simulink model "mod_firmware_NVH_v6"  (R2022a)
settings: Solver=FixedStepDiscrete  StartTime=0.0  StopTime=Inf  RelTol=1e-3  EnableMultiTasking=on
InitFcn:
  | params_NVH;
undefined symbols (not defined in the file): denz, DiscIntNeverNeededParam, Down, GPTRIP1SEL, GPTRIP2SEL, KiTs, Kp, numz, POS, rate_lim, target, Tper, Tref, Ts, TZ1, TZ2, Up
libraries: simulink x10, hdlsllib x7, mcbcontrolslib x5, c2802xlib x4, c2837xDlib x4, c280xlib x2, c2000lib x1, slpidlib x1
(part 1 of 2)
settings Model: ExtModeTrigDuration=8  Creator=Renato  LastModifiedBy=Renato
settings SolverCC: AlgebraicLoopSolver=TrustRegion  AutoInsertRateTranBlk=on
settings OptimizationCC: DefaultUnderspecifiedDataType=single  EnhancedBackFolding=on  PassReuseOutputArgsAs=Individual arguments  MaxStackSize=1024  OptimizeBlockOrder=speed  DifferentSizesBufferReuse=on  OptimizationCustomize=off  DenormalBehavior=FlushToZero  EfficientTunableParamExpr=on
settings DebuggingCC: MultiTaskDSMMsg=none  ParameterPrecisionLossMsg=none  ParameterTunabilityLossMsg=error  UnconnectedInputMsg=warning  UnconnectedOutputMsg=warning  UnconnectedLineMsg=warning  SFMachineParentedDataDiag=warning
settings HardwareCC: ProdBitPerChar=16  ProdBitPerInt=16  ProdBitPerPointer=32  ProdBitPerSizeT=32  ProdBitPerPtrDiffT=32  ProdLargestAtomicInteger=Integer  ProdLargestAtomicFloat=None  ProdWordSize=16  ProdLongLongMode=on  ProdHWDeviceType=Texas Instruments->C2000
settings SFSimCC: MATLABDynamicMemAlloc=off
settings RTWCC: SystemTargetFile=ert.tlc  HardwareBoard=TI Delfino F28379D LaunchPad  TemplateMakefile=ert_default_tmf  Toolchain=Texas Instruments Code Composer Studio (C2000)  DLArmComputeVersion=19.05
settings CodeAppCC: ForceParamTrailComments=on  IgnoreCustomStorageClasses=off  OperatorAnnotations=on  SimulinkDataObjDesc=on  SFDataObjDesc=on  InsertBlockDesc=on
settings ERTTargetCC: CodeReplacementLibrary=TI C28x  ExtModeStaticAllocSize=10000

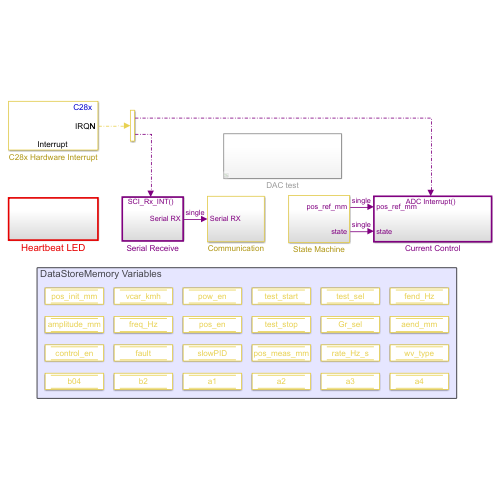
[thumbnail: Simulink's stored preview of the top-level diagram]
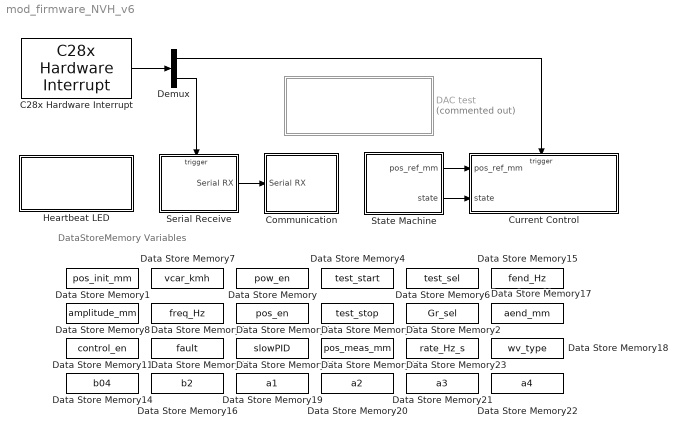
== system mod_firmware_NVH_v6 ==
  note: DataStoreMemory Variables
  C28x Hardware Interrupt : c2000lib/Scheduling/C28x Hardware Interrupt  irqnumbers=[1 9]  pienumbers=[2 1]  irqpriorities=[30 50]  irqpreempts=[1 0]  showinput=off  dspchiptype=C280X
      settings: SourceProductBaseCode=TIC2000
  Communication : Subsystem
  Current Control : Subsystem
  DAC test : Subsystem  Commented=on
  Data Store Memory : DataStoreMemory  DataStoreName=pow_en  ReadBeforeWriteMsg=warning  WriteAfterWriteMsg=warning  WriteAfterReadMsg=warning  ShowAdditionalParam=off
  Data Store Memory1 : DataStoreMemory  DataStoreName=pos_init_mm  ReadBeforeWriteMsg=warning  WriteAfterWriteMsg=warning  WriteAfterReadMsg=warning  ShowAdditionalParam=off
  Data Store Memory10 : DataStoreMemory  DataStoreName=fault  ReadBeforeWriteMsg=warning  WriteAfterWriteMsg=warning  WriteAfterReadMsg=warning  ShowAdditionalParam=off
  Data Store Memory11 : DataStoreMemory  DataStoreName=control_en  ReadBeforeWriteMsg=warning  WriteAfterWriteMsg=warning  WriteAfterReadMsg=warning  ShowAdditionalParam=off
  Data Store Memory12 : DataStoreMemory  DataStoreName=slowPID  ReadBeforeWriteMsg=warning  WriteAfterWriteMsg=warning  WriteAfterReadMsg=warning  ShowAdditionalParam=off
  Data Store Memory13 : DataStoreMemory  DataStoreName=pos_meas_mm  ReadBeforeWriteMsg=warning  WriteAfterWriteMsg=warning  WriteAfterReadMsg=warning  ShowAdditionalParam=off
  Data Store Memory14 : DataStoreMemory  DataStoreName=b04  ReadBeforeWriteMsg=warning  WriteAfterWriteMsg=warning  WriteAfterReadMsg=warning  ShowAdditionalParam=off
  Data Store Memory15 : DataStoreMemory  DataStoreName=fend_Hz  ReadBeforeWriteMsg=warning  WriteAfterWriteMsg=warning  WriteAfterReadMsg=warning  ShowAdditionalParam=off
  Data Store Memory16 : DataStoreMemory  DataStoreName=b2  ReadBeforeWriteMsg=warning  WriteAfterWriteMsg=warning  WriteAfterReadMsg=warning  ShowAdditionalParam=off
  Data Store Memory17 : DataStoreMemory  DataStoreName=aend_mm  ReadBeforeWriteMsg=warning  WriteAfterWriteMsg=warning  WriteAfterReadMsg=warning  ShowAdditionalParam=off
  Data Store Memory18 : DataStoreMemory  DataStoreName=wv_type  ReadBeforeWriteMsg=warning  WriteAfterWriteMsg=warning  WriteAfterReadMsg=warning  ShowAdditionalParam=off
  Data Store Memory19 : DataStoreMemory  DataStoreName=a1  ReadBeforeWriteMsg=warning  WriteAfterWriteMsg=warning  WriteAfterReadMsg=warning  ShowAdditionalParam=off
  Data Store Memory2 : DataStoreMemory  DataStoreName=Gr_sel  ReadBeforeWriteMsg=warning  WriteAfterWriteMsg=warning  WriteAfterReadMsg=warning  ShowAdditionalParam=off
  Data Store Memory20 : DataStoreMemory  DataStoreName=a2  ReadBeforeWriteMsg=warning  WriteAfterWriteMsg=warning  WriteAfterReadMsg=warning  ShowAdditionalParam=off
  Data Store Memory21 : DataStoreMemory  DataStoreName=a3  ReadBeforeWriteMsg=warning  WriteAfterWriteMsg=warning  WriteAfterReadMsg=warning  ShowAdditionalParam=off
  Data Store Memory22 : DataStoreMemory  DataStoreName=a4  ReadBeforeWriteMsg=warning  WriteAfterWriteMsg=warning  WriteAfterReadMsg=warning  ShowAdditionalParam=off
  Data Store Memory23 : DataStoreMemory  DataStoreName=rate_Hz_s  ReadBeforeWriteMsg=warning  WriteAfterWriteMsg=warning  WriteAfterReadMsg=warning  ShowAdditionalParam=off
  Data Store Memory3 : DataStoreMemory  DataStoreName=pos_en  ReadBeforeWriteMsg=warning  WriteAfterWriteMsg=warning  WriteAfterReadMsg=warning  ShowAdditionalParam=off
  Data Store Memory4 : DataStoreMemory  DataStoreName=test_start  ReadBeforeWriteMsg=warning  WriteAfterWriteMsg=warning  WriteAfterReadMsg=warning  ShowAdditionalParam=off
  Data Store Memory5 : DataStoreMemory  DataStoreName=test_stop  ReadBeforeWriteMsg=warning  WriteAfterWriteMsg=warning  WriteAfterReadMsg=warning  ShowAdditionalParam=off
  Data Store Memory6 : DataStoreMemory  DataStoreName=test_sel  ReadBeforeWriteMsg=warning  WriteAfterWriteMsg=warning  WriteAfterReadMsg=warning  ShowAdditionalParam=off
  Data Store Memory7 : DataStoreMemory  DataStoreName=vcar_kmh  ReadBeforeWriteMsg=warning  WriteAfterWriteMsg=warning  WriteAfterReadMsg=warning  ShowAdditionalParam=off
  Data Store Memory8 : DataStoreMemory  DataStoreName=amplitude_mm  ReadBeforeWriteMsg=warning  WriteAfterWriteMsg=warning  WriteAfterReadMsg=warning  ShowAdditionalParam=off
  Data Store Memory9 : DataStoreMemory  DataStoreName=freq_Hz  ReadBeforeWriteMsg=warning  WriteAfterWriteMsg=warning  WriteAfterReadMsg=warning  ShowAdditionalParam=off
  Demux : Demux  Outputs=2
  Heartbeat LED : Subsystem  TreatAsAtomicUnit=on
  Serial Receive : Subsystem  SystemSampleTime=1e-3
  State Machine : Subsystem
  wires:
  C28x Hardware Interrupt/1 -> Demux/1
  Demux/2 -> Serial Receive/Trigger
  Demux/1 -> Current Control/Trigger
  Serial Receive/1(Serial RX) -> Communication/1(Serial RX)
  State Machine/1(pos_ref_mm) -> Current Control/1(pos_ref_mm)
  State Machine/2(state) -> Current Control/2(state)

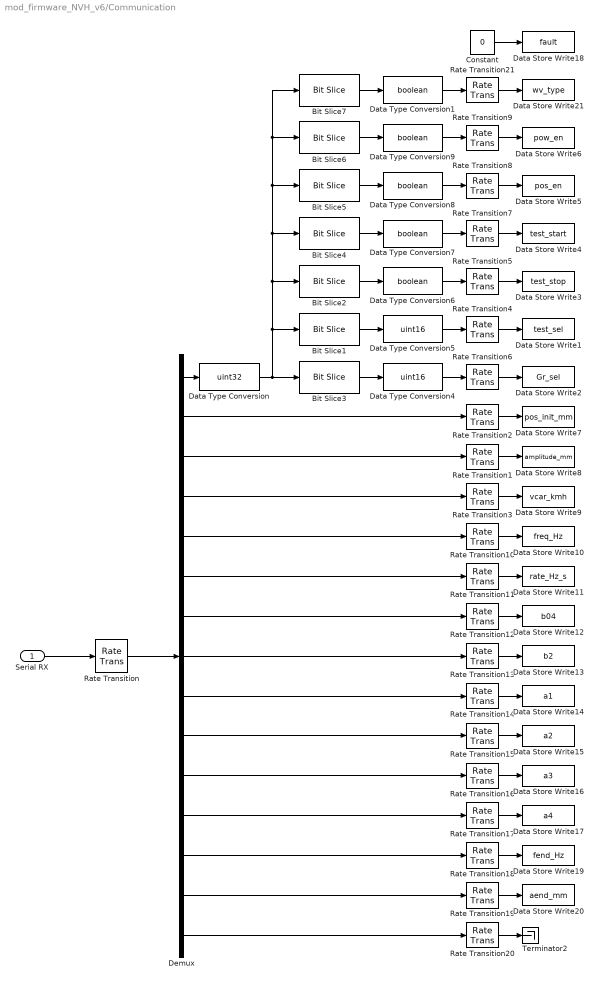
== system mod_firmware_NVH_v6/Communication ==
  Serial RX : Inport
  Bit Slice1 : hdlsllib/Logic and Bit Operations/Bit Slice  lidx=3  ridx=2
      settings: SourceProductBaseCode=SL
  Bit Slice2 : hdlsllib/Logic and Bit Operations/Bit Slice  lidx=4  ridx=4
      settings: SourceProductBaseCode=SL
  Bit Slice3 : hdlsllib/Logic and Bit Operations/Bit Slice  lidx=1  ridx=0
      settings: SourceProductBaseCode=SL
  Bit Slice4 : hdlsllib/Logic and Bit Operations/Bit Slice  lidx=5  ridx=5
      settings: SourceProductBaseCode=SL
  Bit Slice5 : hdlsllib/Logic and Bit Operations/Bit Slice  lidx=6  ridx=6
      settings: SourceProductBaseCode=SL
  Bit Slice6 : hdlsllib/Logic and Bit Operations/Bit Slice  lidx=7  ridx=7
      settings: SourceProductBaseCode=SL
  Bit Slice7 : hdlsllib/Logic and Bit Operations/Bit Slice  lidx=8  ridx=8
      settings: SourceProductBaseCode=SL
  Constant : Constant  Value=0  OutDataTypeStr=boolean  SampleTime=Ts
  Data Store Write1 : DataStoreWrite  DataStoreName=test_sel  IndexOptions=Index vector (dialog)  Indices=1  OutputSizes=1
  Data Store Write10 : DataStoreWrite  DataStoreName=freq_Hz  IndexOptions=Index vector (dialog)  Indices=1  OutputSizes=1
  Data Store Write11 : DataStoreWrite  DataStoreName=rate_Hz_s  IndexOptions=Index vector (dialog)  Indices=1  OutputSizes=1
  Data Store Write12 : DataStoreWrite  DataStoreName=b04  IndexOptions=Index vector (dialog)  Indices=1  OutputSizes=1
  Data Store Write13 : DataStoreWrite  DataStoreName=b2  IndexOptions=Index vector (dialog)  Indices=1  OutputSizes=1
  Data Store Write14 : DataStoreWrite  DataStoreName=a1  IndexOptions=Index vector (dialog)  Indices=1  OutputSizes=1
  Data Store Write15 : DataStoreWrite  DataStoreName=a2  IndexOptions=Index vector (dialog)  Indices=1  OutputSizes=1
  Data Store Write16 : DataStoreWrite  DataStoreName=a3  IndexOptions=Index vector (dialog)  Indices=1  OutputSizes=1
  Data Store Write17 : DataStoreWrite  DataStoreName=a4  IndexOptions=Index vector (dialog)  Indices=1  OutputSizes=1
  Data Store Write18 : DataStoreWrite  DataStoreName=fault  IndexOptions=Index vector (dialog)  Indices=1  OutputSizes=1
  Data Store Write19 : DataStoreWrite  DataStoreName=fend_Hz  IndexOptions=Index vector (dialog)  Indices=1  OutputSizes=1
  Data Store Write2 : DataStoreWrite  DataStoreName=Gr_sel  IndexOptions=Index vector (dialog)  Indices=1  OutputSizes=1
  Data Store Write20 : DataStoreWrite  DataStoreName=aend_mm  IndexOptions=Index vector (dialog)  Indices=1  OutputSizes=1
  Data Store Write21 : DataStoreWrite  DataStoreName=wv_type  IndexOptions=Index vector (dialog)  Indices=1  OutputSizes=1
  Data Store Write3 : DataStoreWrite  DataStoreName=test_stop  IndexOptions=Index vector (dialog)  Indices=1  OutputSizes=1
  Data Store Write4 : DataStoreWrite  DataStoreName=test_start  IndexOptions=Index vector (dialog)  Indices=1  OutputSizes=1
  Data Store Write5 : DataStoreWrite  DataStoreName=pos_en  IndexOptions=Index vector (dialog)  Indices=1  OutputSizes=1
  Data Store Write6 : DataStoreWrite  DataStoreName=pow_en  IndexOptions=Index vector (dialog)  Indices=1  OutputSizes=1
  Data Store Write7 : DataStoreWrite  DataStoreName=pos_init_mm  IndexOptions=Index vector (dialog)  Indices=1  OutputSizes=1
  Data Store Write8 : DataStoreWrite  DataStoreName=amplitude_mm  IndexOptions=Index vector (dialog)  Indices=1  OutputSizes=1
  Data Store Write9 : DataStoreWrite  DataStoreName=vcar_kmh  IndexOptions=Index vector (dialog)  Indices=1  OutputSizes=1
  Data Type Conversion : DataTypeConversion  OutDataTypeStr=uint32  ConvertRealWorld=Stored Integer (SI)  SaturateOnIntegerOverflow=off  RndMeth=Floor
  Data Type Conversion{1,6..9} (5 alike) : DataTypeConversion  OutDataTypeStr=boolean  RndMeth=Simplest  SaturateOnIntegerOverflow=off
  Data Type Conversion4 : DataTypeConversion  OutDataTypeStr=uint16  RndMeth=Simplest  SaturateOnIntegerOverflow=off
  Data Type Conversion5 : DataTypeConversion  OutDataTypeStr=uint16  RndMeth=Simplest  SaturateOnIntegerOverflow=off
  Demux : Demux  Outputs=15
  Rate Transition : RateTransition  Deterministic=off  InitialCondition=zeros(15,1)  OutPortSampleTime=Ts
  Rate Transition{1..21} (21 alike) : RateTransition  Deterministic=off
  Terminator2 : Terminator
  wires:
  Rate Transition/1 -> Demux/1
  Serial RX/1 -> Rate Transition/1
  Demux/1 -> Data Type Conversion/1
  Bit Slice3/1 -> Data Type Conversion4/1
  Data Type Conversion4/1 -> Rate Transition6/1
  Bit Slice1/1 -> Data Type Conversion5/1
  Data Type Conversion5/1 -> Rate Transition4/1
  Data Type Conversion6/1 -> Rate Transition5/1
  Bit Slice2/1 -> Data Type Conversion6/1
  Data Type Conversion7/1 -> Rate Transition7/1
  Bit Slice4/1 -> Data Type Conversion7/1
  Data Type Conversion8/1 -> Rate Transition8/1
  Bit Slice5/1 -> Data Type Conversion8/1
  Data Type Conversion9/1 -> Rate Transition9/1
  Bit Slice6/1 -> Data Type Conversion9/1
  Rate Transition6/1 -> Data Store Write2/1
  Rate Transition4/1 -> Data Store Write1/1
  Rate Transition5/1 -> Data Store Write3/1
  Rate Transition7/1 -> Data Store Write4/1
  Rate Transition8/1 -> Data Store Write5/1
  Rate Transition9/1 -> Data Store Write6/1
  Demux/2 -> Rate Transition2/1
  Rate Transition2/1 -> Data Store Write7/1
  Rate Transition1/1 -> Data Store Write8/1
  Demux/3 -> Rate Transition1/1
  Rate Transition3/1 -> Data Store Write9/1
  Demux/4 -> Rate Transition3/1
  Demux/5 -> Rate Transition10/1
  Rate Transition10/1 -> Data Store Write10/1
  Constant/1 -> Data Store Write18/1
  Rate Transition20/1 -> Terminator2/1
  Rate Transition19/1 -> Data Store Write20/1
  Rate Transition18/1 -> Data Store Write19/1
  Rate Transition17/1 -> Data Store Write17/1
  Demux/6 -> Rate Transition11/1
  Rate Transition11/1 -> Data Store Write11/1
  Rate Transition13/1 -> Data Store Write13/1
  Rate Transition15/1 -> Data Store Write15/1
  Rate Transition12/1 -> Data Store Write12/1
  Rate Transition14/1 -> Data Store Write14/1
  Rate Transition16/1 -> Data Store Write16/1
  Demux/7 -> Rate Transition12/1
  Demux/8 -> Rate Transition13/1
  Demux/9 -> Rate Transition14/1
  Demux/10 -> Rate Transition15/1
  Demux/11 -> Rate Transition16/1
  Demux/14 -> Rate Transition19/1
  Demux/12 -> Rate Transition17/1
  Demux/15 -> Rate Transition20/1
  Demux/13 -> Rate Transition18/1
  Data Type Conversion/1 -> Bit Slice5/1, Bit Slice7/1, Bit Slice6/1, Bit Slice4/1, Bit Slice2/1, Bit Slice1/1, Bit Slice3/1
  Rate Transition21/1 -> Data Store Write21/1
  Data Type Conversion1/1 -> Rate Transition21/1
  Bit Slice7/1 -> Data Type Conversion1/1

== system mod_firmware_NVH_v6/Current Control ==
  pos_ref_mm : Inport
  state : Inport  Port=2
  ADC Interrupt : TriggerPort  TriggerType=function-call  VariantControl=Variant
  ADC sampling : Subsystem
      settings: PortSchema="{\"entries\":[{\"content\":{\"sides\":[{\"content\":{\"connectorIds\":[]},\"type\":\"ConnectorPlacement.EquallySpacedRectSide\",\"uuid\":\"7a2cf5f2-16d9-4c06-9e50-766569fc1ffb\"},{\"content\":{\"connectorIds\":[],\"side\":\"RIGHT\"},\"type\":\"ConnectorPlacement.EquallySpacedRectSide\",\"uuid\":\"bcd2dcb7-1f81-4f8a-ab4d-3b7c4b9f9b31\"},{\"content\":{\"connectorIds\":[\"Out1\",\"In1\"],\"side\":\"TOP\"},\"type\":\"ConnectorPlacement.EquallySpacedRectSide\",\"uuid\":\"ccc507c4-0562-40ca-8656-7bb2ecd7cc5f\"}]},\"type\":\"ConnectorPlacement.EquallySpacedConnector\",\"uuid\":\"1a99524b-495c-42f0-b183-14d68da7a393\"}],\"packageUris\":[\"http://schema.mathworks.com/mf0/Connector/R2020b\"],\"version\":\"1.0\"}"
  Data Serial Output : Subsystem
  Duty conditioning : Subsystem
      settings: PortSchema="{\"entries\":[{\"content\":{\"sides\":[{\"content\":{\"connectorIds\":[\"In1\"]},\"type\":\"ConnectorPlacement.EquallySpacedRectSide\",\"uuid\":\"a0799500-10a4-4433-8e57-709958199fd5\"},{\"content\":{\"connectorIds\":[\"Out1\",\"In2\"],\"side\":\"RIGHT\"},\"type\":\"ConnectorPlacement.EquallySpacedRectSide\",\"uuid\":\"3bf72f91-b298-49c1-8116-d920c6c6ec77\"},{\"content\":{\"connectorIds\":[],\"side\":\"TOP\"},\"type\":\"ConnectorPlacement.EquallySpacedRectSide\",\"uuid\":\"802670f8-b9dd-4762-928c-43325713460b\"}]},\"type\":\"ConnectorPlacement.EquallySpacedConnector\",\"uuid\":\"a1eb57ea-35c4-47bc-baa8-d00685cc87f7\"}],\"packageUris\":[\"http://schema.mathworks.com/mf0/Connector/R2020b\"],\"version\":\"1.0\"}"
  Hardware Initialization : Subsystem
  Mux : Mux  Inputs=3
  PWM : Subsystem
  wires:
  Duty conditioning/1(dutyA) -> PWM/1(dutyA), ADC sampling/1(dutyA)
  Mux/1 -> Data Serial Output/1(send_vec)
  state/1 -> Mux/3
  pos_ref_mm/1 -> Mux/1, Duty conditioning/1(pos_ref_mm)
  ADC sampling/1(pos_meas) -> Duty conditioning/2(pos_meas), Mux/2

== system mod_firmware_NVH_v6/DAC test ==
  DAC : c2837xDlib/DAC  channel=B  saturate=on
      settings: SourceProductBaseCode=TIC2000
  Data Type Conversion : DataTypeConversion  OutDataTypeStr=uint16  SaturateOnIntegerOverflow=off  RndMeth=Floor
  Sine Wave : Sin  Amplitude=2048-100  Bias=2048  Frequency=2*pi  SampleTime=Ts
  Sine Wave1 : Sin  Amplitude=100  Frequency=2*pi*2000  SampleTime=Ts
  Sum : Sum  Inputs=|++
  wires:
  Data Type Conversion/1 -> DAC/1
  Sum/1 -> Data Type Conversion/1
  Sine Wave/1 -> Sum/1
  Sine Wave1/1 -> Sum/2

== system mod_firmware_NVH_v6/Heartbeat LED ==
  Data Store Read1 : DataStoreRead  DataStoreName=pos_en  IndexOptions=Index vector (dialog)  Indices=1  OutputSizes=1
  Digital Output : c2837xDlib/Digital Output  GPIO_Number=GPIO32~GPIO39  GPIO_Bit0=off  GPIO_BIT0_Toggle=on  GPIO_Bit1=off  GPIO_BIT1_Toggle=off  GPIO_Bit2=on  GPIO_BIT2_Toggle=off  GPIO_Bit3=off  GPIO_BIT3_Toggle=off  GPIO_Bit4=off  GPIO_BIT4_Toggle=off  GPIO_Bit5=off  GPIO_BIT5_Toggle=off  GPIO_Bit6=off  GPIO_BIT6_Toggle=off  GPIO_Bit7=off  GPIO_BIT7_Toggle=off
      settings: SourceProductBaseCode=TIC2000
  wires:
  Data Store Read1/1 -> Digital Output/1

== system mod_firmware_NVH_v6/Serial Receive ==
  SCI_Rx_INT : TriggerPort  TriggerType=function-call  VariantControl=Variant
  SCI Receive : c280xlib/SCI Receive  sciModule=A  dataHead=''  headerCheckMaxCount=16  dataTail=''  dataType=single  dataLenOptions=Length via dialog  dataDim=15  maxDataLength=1  initValue=0  errOption=Output the last received value  errValue=0  sampleTime=-1  blockingMode=on  timeOut=0.00875  outputStatus=off
      settings: SourceProductBaseCode=TIC2000
  Serial RX : Outport  VectorParamsAs1DForOutWhenUnconnected=off
  wires:
  SCI Receive/1 -> Serial RX/1

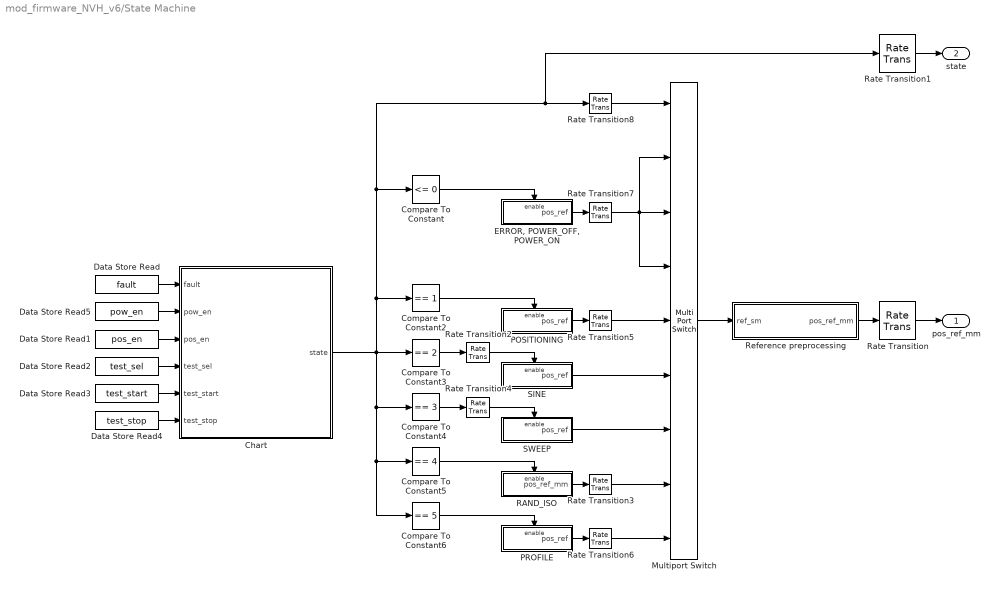
== system mod_firmware_NVH_v6/State Machine ==
  Chart : Stateflow chart  TreatAsAtomicUnit=on
  Compare To Constant : simulink/Logic and Bit Operations/Compare To Constant  relop=<=  const=0  OutDataTypeStr=boolean
  Compare To Constant2 : simulink/Logic and Bit Operations/Compare To Constant  relop===  const=1  OutDataTypeStr=boolean
  Compare To Constant3 : simulink/Logic and Bit Operations/Compare To Constant  relop===  const=2  OutDataTypeStr=boolean
  Compare To Constant4 : simulink/Logic and Bit Operations/Compare To Constant  relop===  const=3  OutDataTypeStr=boolean
  Compare To Constant5 : simulink/Logic and Bit Operations/Compare To Constant  relop===  const=4  OutDataTypeStr=boolean
  Compare To Constant6 : simulink/Logic and Bit Operations/Compare To Constant  relop===  const=5  OutDataTypeStr=boolean
  Data Store Read : DataStoreRead  DataStoreName=fault  SampleTime=Tref  IndexOptions=Index vector (dialog)  Indices=1  OutputSizes=1
  Data Store Read1 : DataStoreRead  DataStoreName=pos_en  SampleTime=Tref  IndexOptions=Index vector (dialog)  Indices=1  OutputSizes=1
  Data Store Read2 : DataStoreRead  DataStoreName=test_sel  SampleTime=Tref  IndexOptions=Index vector (dialog)  Indices=1  OutputSizes=1
  Data Store Read3 : DataStoreRead  DataStoreName=test_start  SampleTime=Tref  IndexOptions=Index vector (dialog)  Indices=1  OutputSizes=1
  Data Store Read4 : DataStoreRead  DataStoreName=test_stop  SampleTime=Tref  IndexOptions=Index vector (dialog)  Indices=1  OutputSizes=1
  Data Store Read5 : DataStoreRead  DataStoreName=pow_en  SampleTime=Tref  IndexOptions=Index vector (dialog)  Indices=1  OutputSizes=1
  "ERROR, POWER_OFF, POWER_ON" : Subsystem  TreatAsAtomicUnit=on
  Multiport Switch : MultiPortSwitch  DataPortOrder=Specify indices  Inputs=7  DataPortIndices={-2,-1,0,1,2,3,4,5}  SaturateOnIntegerOverflow=off  InputSameDT=off
  POSITIONING : Subsystem  TreatAsAtomicUnit=on
  PROFILE : Subsystem  TreatAsAtomicUnit=on
  RAND_ISO : Subsystem  TreatAsAtomicUnit=on
  Rate Transition : RateTransition  Deterministic=off
  Rate Transition1 : RateTransition  Deterministic=off
  Rate Transition{2..8} (7 alike) : RateTransition  Deterministic=off  OutPortSampleTime=Tper
  Reference preprocessing : Subsystem
  SINE : Subsystem  TreatAsAtomicUnit=on
  SWEEP : Subsystem  TreatAsAtomicUnit=on
  pos_ref_mm : Outport
  state : Outport  Port=2
  wires:
  Data Store Read3/1 -> Chart/5(test_start)
  Data Store Read2/1 -> Chart/4(test_sel)
  Data Store Read/1 -> Chart/1(fault)
  Data Store Read1/1 -> Chart/3(pos_en)
  Data Store Read4/1 -> Chart/6(test_stop)
  Compare To Constant/1 -> "ERROR, POWER_OFF, POWER_ON"/Enable
  "ERROR, POWER_OFF, POWER_ON"/1(pos_ref) -> Rate Transition7/1
  Compare To Constant2/1 -> POSITIONING/Enable
  Compare To Constant6/1 -> PROFILE/Enable
  Compare To Constant5/1 -> RAND_ISO/Enable
  Compare To Constant4/1 -> Rate Transition4/1
  Compare To Constant3/1 -> Rate Transition2/1
  Rate Transition1/1 -> state/1
  Rate Transition/1 -> pos_ref_mm/1
  Chart/1(state) -> Rate Transition1/1, Rate Transition8/1, Compare To Constant/1, Compare To Constant2/1, Compare To Constant4/1, Compare To Constant6/1, Compare To Constant5/1, Compare To Constant3/1
  Data Store Read5/1 -> Chart/2(pow_en)
  POSITIONING/1(pos_ref) -> Rate Transition5/1
  RAND_ISO/1(pos_ref_mm) -> Rate Transition3/1
  PROFILE/1(pos_ref) -> Rate Transition6/1
  Multiport Switch/1 -> Reference preprocessing/1(ref_sm)
  Reference preprocessing/1(pos_ref_mm) -> Rate Transition/1
  Rate Transition2/1 -> SINE/Enable
  SINE/1(pos_ref) -> Multiport Switch/6
  Rate Transition4/1 -> SWEEP/Enable
  SWEEP/1(pos_ref) -> Multiport Switch/7
  Rate Transition6/1 -> Multiport Switch/9
  Rate Transition3/1 -> Multiport Switch/8
  Rate Transition5/1 -> Multiport Switch/5
  Rate Transition7/1 -> Multiport Switch/4, Multiport Switch/2, Multiport Switch/3
  Rate Transition8/1 -> Multiport Switch/1

== system mod_firmware_NVH_v6/Current Control/ADC sampling ==
  dutyA : Inport
  Convert : Subsystem
  H1-J7 64 : c2802xlib/ADC  blkParamProc=C2000_Type4  ADCModule=C  samplingMode=Single sample mode  ADCResolution=12-bit (Single-ended input)  useSOC1=SOC1  useSOC2=SOC0_SOC1  SOCAcquisitionWindow=300  SOCTriggerSource=ePWM1_ADCSOCA  SOCInterruptTrigger=No ADCINT  Ts=-1  dType=uint16  postInterrupt=off  interruptSel=ADCINT1  ADCINTContinuous=on  endma=off  chdma=1  conv1=ADCINA0  conv2=ADCINA0 and ADCINB0  conv1_Type4=ADCIN5  conv2_Type4=ADCIN0 and ADCIN1
  IIR Filter : mcbcontrolslib/IIR Filter  VariantControl=Low Pass Filter  VariantSelect=Low-pass  Filter_constant=0.12  advancedSettings=on  Ts=Ts  cutOff_freq=434.0589
      settings: SourceProductBaseCode=MT
  ISENA : c2802xlib/ADC  blkParamProc=C2000_Type4  ADCModule=B  samplingMode=Single sample mode  ADCResolution=12-bit (Single-ended input)  useSOC1=SOC0  useSOC2=SOC0_SOC1  SOCAcquisitionWindow=300  SOCTriggerSource=ePWM1_ADCSOCA  SOCInterruptTrigger=No ADCINT  Ts=-1  dType=uint16  postInterrupt=on  interruptSel=ADCINT1  ADCINTContinuous=on  endma=off  chdma=1  conv1=ADCINA0  conv2=ADCINA0 and ADCINB0  conv1_Type4=ADCIN2  conv2_Type4=ADCIN0 and ADCIN1
  Terminator : Terminator
  Terminator1 : Terminator
  pos_meas : Outport  InitialOutput=0  VectorParamsAs1DForOutWhenUnconnected=off
  wires:
  H1-J7 64/1 -> Convert/1(ADC)
  dutyA/1 -> Terminator/1
  ISENA/1 -> Terminator1/1
  Convert/1(mm) -> IIR Filter/1
  IIR Filter/1 -> pos_meas/1

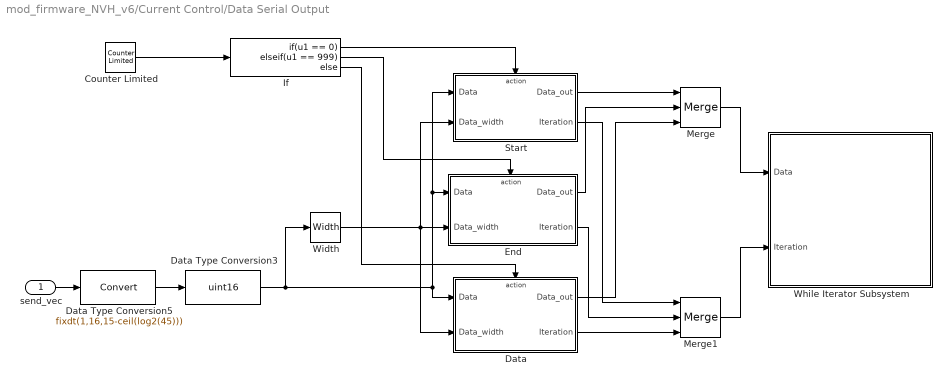
== system mod_firmware_NVH_v6/Current Control/Data Serial Output ==
  send_vec : Inport
  Counter Limited : simulink/Sources/Counter Limited  uplimit=999  tsamp=-1
  Data : Subsystem  TreatAsAtomicUnit=on
  Data Type Conversion3 : DataTypeConversion  OutDataTypeStr=uint16  ConvertRealWorld=Stored Integer (SI)  SaturateOnIntegerOverflow=off  RndMeth=Floor
  Data Type Conversion5 : DataTypeConversion  OutDataTypeStr=fixdt(1,16,15-ceil(log2(45)))  RndMeth=Simplest  SaturateOnIntegerOverflow=off
  End : Subsystem  TreatAsAtomicUnit=on
  If : If  IfExpression=u1 == 0  ElseIfExpressions=u1 == 999
  Merge : Merge  Inputs=3
  Merge1 : Merge  Inputs=3
  Start : Subsystem  TreatAsAtomicUnit=on
  While Iterator Subsystem : Subsystem  TreatAsAtomicUnit=on
  Width : Width  OutDataTypeMode=All ports same datatype  DataType=uint16
  wires:
  Merge/1 -> While Iterator Subsystem/1(Data)
  If/2 -> End/Action
  If/3 -> Data/Action
  Counter Limited/1 -> If/1
  End/1(Data_out) -> Merge/2
  Width/1 -> Start/2(Data_width), Data/2(Data_width), End/2(Data_width)
  Start/1(Data_out) -> Merge/1
  Start/2(Iteration) -> Merge1/1
  Merge1/1 -> While Iterator Subsystem/2(Iteration)
  Data/1(Data_out) -> Merge/3
  If/1 -> Start/Action
  End/2(Iteration) -> Merge1/2
  Data/2(Iteration) -> Merge1/3
  Data Type Conversion3/1 -> Width/1, Start/1(Data), End/1(Data), Data/1(Data)
  send_vec/1 -> Data Type Conversion5/1
  Data Type Conversion5/1 -> Data Type Conversion3/1

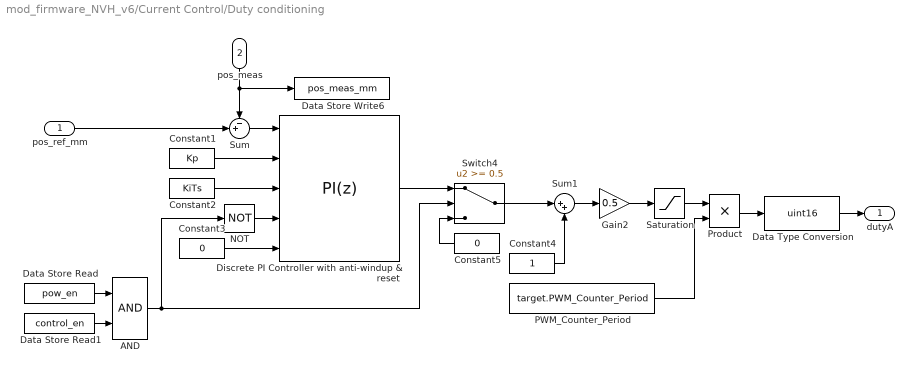
== system mod_firmware_NVH_v6/Current Control/Duty conditioning ==
  pos_ref_mm : Inport
  pos_meas : Inport  Port=2
  AND : Logic  IconShape=distinctive  AllPortsSameDT=off  OutDataTypeStr=boolean
  Constant1 : Constant  Value=Kp  OutDataTypeStr=dataType  SampleTime=-1
  Constant2 : Constant  Value=KiTs  OutDataTypeStr=dataType  SampleTime=-1
  Constant3 : Constant  Value=0  OutDataTypeStr=dataType  SampleTime=-1
  Constant4 : Constant  OutDataTypeStr=dataType  SampleTime=-1
  Constant5 : Constant  Value=0  OutDataTypeStr=dataType  SampleTime=-1
  Data Store Read : DataStoreRead  DataStoreName=pow_en  IndexOptions=Index vector (dialog)  Indices=1  OutputSizes=1
  Data Store Read1 : DataStoreRead  DataStoreName=control_en  IndexOptions=Index vector (dialog)  Indices=1  OutputSizes=1
  Data Store Write6 : DataStoreWrite  DataStoreName=pos_meas_mm  IndexOptions=Index vector (dialog)  Indices=1  OutputSizes=1
  Data Type Conversion : DataTypeConversion  OutDataTypeStr=uint16  RndMeth=Simplest
  Discrete PI Controller with anti-windup & reset : slpidlib/PID Controller  Controller=PI  Form=Parallel  TimeDomain=Discrete-time  UseExternalTs=off  SampleTime=-1  IntegratorMethod=Forward Euler  FilterMethod=Forward Euler  ControllerParametersSource=external  P=1  I=1  UseKiTs=on  D=0  N=100  UseFilter=on  TunerSelectOption=Transfer Function Based (PID Tuner App)  InitialConditionSource=external  InitialConditionForIntegrator=0  InitialConditionForFilter=0  DifferentiatorICPrevScaledInput=0  ExternalReset=level  TrackingMode=off  Kt=1  LimitOutput=on  SatLimitsSource=internal  UpperSaturationLimit=1  LowerSaturationLimit=-1  LinearizeAsGain=on  AntiWindupMode=clamping  Kb=1  RndMeth=Simplest  POutMin=[]  POutMax=[]  IOutMin=[]  IOutMax=[]  DOutMin=[]  DOutMax=[]  NOutMin=[]  NOutMax=[]  SumOutMin=[]  SumOutMax=[]  SaturationOutDataTypeStr=Inherit: Inherit via back propagation  SaturationOutMin=[]  SaturationOutMax=[]  PParamMin=[]  PParamMax=[]  IParamMin=[]  IParamMax=[]  DParamMin=[]  DParamMax=[]  NParamMin=[]  NParamMax=[]  KbParamMin=[]  KbParamMax=[]  KtParamMin=[]  KtParamMax=[]  KbOutMin=[]  KbOutMax=[]  KtOutMin=[]  KtOutMax=[]  IntegratorOutMin=[]  IntegratorOutMax=[]  FilterOutMin=[]  FilterOutMax=[]  SumI1OutMin=[]  SumI1OutMax=[]  SumI2OutMin=[]  SumI2OutMax=[]  SumI3OutMin=[]  SumI3OutMax=[]  SumI4OutMin=[]  SumI4OutMax=[]  SumDOutMin=[]  SumDOutMax=[]  DifferentiatorOutMin=[]  DifferentiatorOutMax=[]  FilterDiffOutCoefMin=[]  FilterDiffOutCoefMax=[]  ReciprocalOutMin=[]  ReciprocalOutMax=[]  SumDenOutMin=[]  SumDenOutMax=[]  SumNumOutMin=[]  SumNumOutMax=[]  DivideOutMin=[]  DivideOutMax=[]  UdiffTsProdOutMin=[]  UdiffTsProdOutMax=[]  NTsProdOutMin=[]  NTsProdOutMax=[]  UintegralTsProdOutMin=[]  UintegralTsProdOutMax=[]  UngainTsProdOutMin=[]  UngainTsProdOutMax=[]  ClampingZeroOutDataTypeStr=Inherit: Inherit via back propagation  ClampingZeroOutMin=[]  ClampingZeroOutMax=[]  FilterDenConstantOutDataTypeStr=Inherit: Inherit via back propagation  FilterDenConstantOutMin=[]  FilterDenConstantOutMax=[]  PCopyOutDataTypeStr=Inherit: Inherit via back propagation  PCopyOutMin=[]  PCopyOutMax=[]  NCopyOutDataTypeStr=Inherit: Inherit via back propagation  NCopyOutMin=[]  NCopyOutMax=[]  IntegratorContinuousStateAttributes=''  IntegratorStateMustResolveToSignalObject=off  IntegratorRTWStateStorageClass=Auto  FilterContinuousStateAttributes=''  FilterStateMustResolveToSignalObject=off  FilterRTWStateStorageClass=Auto  ParallelPVariant=ExternalParameters  IdealPVariant=Disabled  IVariant=ExternalParameters  DVariant=Disabled  IntegratorVariant=Discrete  SatVariant=Enabled  AWVariant=DiscClampingParallel  PCopyVariant=Disabled  TRVariant=Disabled  FdbkBlocksVariant=Forward  IdealPFdbkVariant=Disabled  SatFdbkVariant=Disabled  DerivativeFilterVariant=Disabled  NVariant=Disabled  NCopyVariant=Disabled_SignalSpec  FilterICVariant=Disabled  IntegratorICVariant=ExternalICs  ExternalResetVariant=ExternalReset  TRSumVariant=Passthrough  SumFdbkVariant=Disabled  SumVariant=Sum_PI  TsampFilterVariant=InternalTs  TsampNgainVariant=Passthrough  TsampIntegralVariant=Passthrough  ExternalSaturationOutDataTypeStr=Inherit: Same as second input  aMode=5
  Gain2 : Gain  Gain=0.5  OutDataTypeStr=dataType  RndMeth=Simplest
  NOT : Logic  Operator=NOT  IconShape=distinctive  AllPortsSameDT=off  OutDataTypeStr=boolean
  PWM_Counter_Period : Constant  Value=target.PWM_Counter_Period  OutDataTypeStr=dataType  SampleTime=-1
  Product : Product  RndMeth=Simplest  OutDataTypeStr=Inherit: Same as first input
  Saturation : Saturate  UpperLimit=0.71  LowerLimit=0.29  RndMeth=Simplest
  Sum : Sum  Inputs=-+|
  Sum1 : Sum  Inputs=|++
  Switch4 : Switch  Threshold=0.5  RndMeth=Simplest  SaturateOnIntegerOverflow=off  InputSameDT=off
  dutyA : Outport
  wires:
  Product/1 -> Data Type Conversion/1
  PWM_Counter_Period/1 -> Product/2
  Data Type Conversion/1 -> dutyA/1
  pos_ref_mm/1 -> Sum/2
  pos_meas/1 -> Data Store Write6/1, Sum/1
  Sum/1 -> Discrete PI Controller with anti-windup & reset/1
  Constant4/1 -> Sum1/2
  Sum1/1 -> Gain2/1
  Gain2/1 -> Saturation/1
  Saturation/1 -> Product/1
  AND/1 -> NOT/1, Switch4/2
  NOT/1 -> Discrete PI Controller with anti-windup & reset/4
  Constant3/1 -> Discrete PI Controller with anti-windup & reset/5
  Discrete PI Controller with anti-windup & reset/1 -> Switch4/1
  Switch4/1 -> Sum1/1
  Constant5/1 -> Switch4/3
  Data Store Read/1 -> AND/1
  Data Store Read1/1 -> AND/2
  Constant1/1 -> Discrete PI Controller with anti-windup & reset/2
  Constant2/1 -> Discrete PI Controller with anti-windup & reset/3

== system mod_firmware_NVH_v6/Current Control/Hardware Initialization ==
  " Grounding the SPI clock for the DRV8323" : c2837xDlib/Digital Output  GPIO_Number=GPIO56~GPIO63  GPIO_Bit0=off  GPIO_BIT0_Toggle=off  GPIO_Bit1=off  GPIO_BIT1_Toggle=off  GPIO_Bit2=off  GPIO_BIT2_Toggle=off  GPIO_Bit3=off  GPIO_BIT3_Toggle=off  GPIO_Bit4=on  GPIO_BIT4_Toggle=off  GPIO_Bit5=off  GPIO_BIT5_Toggle=off  GPIO_Bit6=off  GPIO_BIT6_Toggle=off  GPIO_Bit7=off  GPIO_BIT7_Toggle=off
      settings: SourceProductBaseCode=TIC2000
  Constant : Constant  Value=0  OutDataTypeStr=uint16  SampleTime=-1
  DRV8323 Enable : c2837xDlib/Digital Output  GPIO_Number=GPIO64~GPIO71  GPIO_Bit0=off  GPIO_BIT0_Toggle=off  GPIO_Bit1=off  GPIO_BIT1_Toggle=off  GPIO_Bit2=off  GPIO_BIT2_Toggle=off  GPIO_Bit3=on  GPIO_BIT3_Toggle=off  GPIO_Bit4=off  GPIO_BIT4_Toggle=off  GPIO_Bit5=off  GPIO_BIT5_Toggle=off  GPIO_Bit6=off  GPIO_BIT6_Toggle=off  GPIO_Bit7=off  GPIO_BIT7_Toggle=off
      settings: SourceProductBaseCode=TIC2000
  Data Store Read : DataStoreRead  DataStoreName=pow_en  IndexOptions=Index vector (dialog)  Indices=1  OutputSizes=1
  wires:
  Constant/1 -> " Grounding the SPI clock for the DRV8323"/1
  Data Store Read/1 -> DRV8323 Enable/1

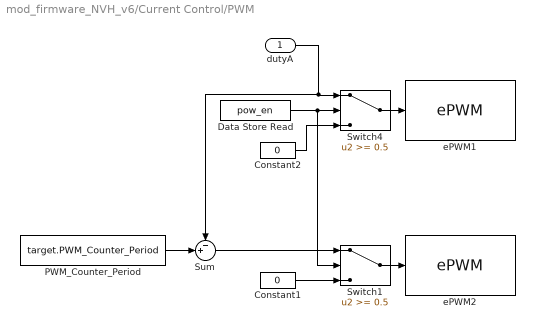
== system mod_firmware_NVH_v6/Current Control/PWM ==
  dutyA : Inport
  Constant1 : Constant  Value=0  OutDataTypeStr=uint16
  Constant2 : Constant  Value=0  OutDataTypeStr=uint16
  Data Store Read : DataStoreRead  DataStoreName=pow_en  IndexOptions=Index vector (dialog)  Indices=1  OutputSizes=1
  PWM_Counter_Period : Constant  Value=target.PWM_Counter_Period  OutDataTypeStr=uint16  SampleTime=-1
  Sum : Sum  Inputs=-+|
  Switch1 : Switch  Threshold=0.5  RndMeth=Simplest  SaturateOnIntegerOverflow=off  InputSameDT=off
  Switch4 : Switch  Threshold=0.5  RndMeth=Simplest  SaturateOnIntegerOverflow=off  InputSameDT=off
  ePWM1 : c2802xlib/ePWM  PwmType=C2000_Type4  useModule=ePWM1  ePWMxLINKTBPRD=Not Linked  periodUnits=Clock cycles  timerSource=Specify via dialog  timerPeriod_clk=target.PWM_Counter_Period+1  timerPeriod_sec=0.0001  tbshadow=Counter equals to zero  countingMode=Up-Down  phaseActiveEnable=Disable  phaseDirection=Count down after sync  phaseActive=0  synchronizationEnable=off  dcaevt1Sync=off  dcbevt1Sync=off  synchronizationOption=Counter equals to zero (CTR=Zero)  perSynchronizationOption=Counter equals to period (CTR=PRD)  clockPrescale=1  HSclockPrescale=1  enswap=off  ePWMxAStatus=on  ePWMxAactionLogic1=Do nothing  ePWMxAactionLogic2=Do nothing  ePWMxAactionLogic3=Clear  ePWMxAactionLogic4=Set  ePWMxAactionLogic5=Do nothing  ePWMxAactionLogic6=Do nothing  ePWMxACSFenable=off  ePWMxACSFvalue=Forcing disable  ePWMxASFreload=Zero  ePWMxBStatus=off  ePWMxBactionLogic1=Set  ePWMxBactionLogic2=Clear  ePWMxBactionLogic3=Do nothing  ePWMxBactionLogic4=Do nothing  ePWMxBactionLogic5=Clear  ePWMxBactionLogic6=Set  ePWMxBCSFenable=off  ePWMxBCSFvalue=Forcing disable  ePWMxBSFreload=Zero  ePWNxBOutWay=off  ePWMxLINKCMPA=Not Linked  CMPAUnits=Clock cycles  CMPASource=Input port  CMPAValue_per=50  CMPAValue_clk=floor(target.PWM_Counter_Period/2+1)  enCMPAshadow=Counter equals to zero (CTR=Zero)  ePWMxLINKCMPB=Not Linked  CMPBUnits=Clock cycles  CMPBSource=Specify via dialog  CMPBValue_per=50  CMPBValue_clk=floor(target.PWM_Counter_Period/2+1)  enCMPBshadow=Counter equals to zero (CTR=Zero)  ePWMxLINKCMPC=Not Linked  CMPCUnits=Clock cycles  CMPCSource=Specify via dialog  CMPCValue_per=50  CMPCValue_clk=32000  enCMPCshadow=Counter equals to zero (CTR=Zero)  ePWMxLINKCMPD=Not Linked  CMPDUnits=Clock cycles  CMPDSource=Specify via dialog  CMPDValue_per=50  CMPDValue_clk=32000  enCMPDshadow=Counter equals to zero (CTR=Zero)  enableDBePWMxA=on  enableDBePWMxB=on  enhalfcycle=off  DBpolarity=Active high complementary (AHC)  DBedgeDelay=Positive  DBSource_ePWMxA=ePWMxA  DBSource_ePWMxB=ePWMxA  DBPeriodUnits=Clock cycles  DBperiodSource=Specify via dialog  REDperiod=15  FEDperiod=15  REDperiod_sec=0  FEDperiod_sec=0  LoadModeDBRED=Immediate without using shadow  LoadModeDBFED=Immediate without using shadow  adcstartModuleA=on  adcrequestEventA=First event  adcstartEventA=Digital Compare Module A Event 1 start of conversion (DCAEVT1.soc)  adcstartEventA_type2=Counter equals to period (CTR=PRD)  adcstartModuleB=off  adcrequestEventB=First event  adcstartEventB=Counter equals to zero (CTR=Zero)  adcstartEventB_type2=Counter equals to zero (CTR=Zero)  intEn=off  intPrd=First event  intSel=Counter equals to zero (CTR=Zero)  intSel_type2=Counter equals to zero (CTR=Zero)  hrpe=off  enHRPWM=off  HRPWM_LoadMode=Counter equals to period (CTR=PRD)  HRPWM_CTLMode=Duty or Period control mode  HRPWM_EDGMode=Both edge  hrpeb=off  enHRPWMB=off  HRPWM_LoadModeB=Counter equals to zero (CTR=ZERO)  HRPWM_CTLModeB=Duty or Period control mode  HRPWM_EDGModeB=Both edge  enHRDBRED=off  enHRDBFED=off  enSFO=on  enautoconv=on  chopperEnable=off  chopperFrequency=1  chopperFirstwidth=1  chopperDuty=12.5%  tripZonesource=Specify via dialog  tzselOSHT1=off  tzselOSHT2=off  tzselOSHT3=off  tzselOSHDCAEV1=off  tzselOSHDCBEV1=off  tzselCBC1=off  tzselCBC2=off  tzselCBC3=off  tzselCBCDCAEV2=off  tzselCBCDCBEV2=off  tzselOSHT4=off  tzselOSHT5=off  tzselOSHT6=off  tzselCBC4=off  tzselCBC5=off  tzselCBC6=off  enTzOstIntr=off  enTzCbcIntr=off  enTzDCAEVT1Intr=off  enTzDCAEVT2Intr=off  enTzDCBEVT1Intr=off  enTzDCBEVT2Intr=off  ePWMxAforced=No action  ePWMxBforced=No action  DCAEVT1forced=No action  DCBEVT1forced=No action  DCAEVT2forced=No action  DCBEVT2forced=No action  dcah=Trip Zone 1 input (TZ1)  dcal=Trip Zone 2 input (TZ2)  dcbh=Trip Zone 1 input (TZ1)  dcbl=Trip Zone 2 input (TZ2)  dcah_type2=GPTRIP1SEL/(TZ1)  dcal_type2=GPTRIP2SEL/(TZ2)  dcbh_type2=GPTRIP1SEL/(TZ1)  dcbl_type2=GPTRIP2SEL/(TZ2)  gendcaevt1=Event disabled  gendcaevt2=Event disabled  gendcbevt1=Event disabled  gendcbevt2=Event disabled  dcaevt1src=DCAEVT1 with sync  dcaevt2src=DCAEVT2 with sync  dcbevt1src=DCBEVT1 with sync  dcbevt2src=DCBEVT2 with sync  pulsesel=Counter equals to zero (CTR=Zero)  blankinv=off  blankoffset=0  blankwidth=0  evsrcsel=Filtered version of DCAEVT1 (DCAEVT1FILT)  encape=off
  ePWM2 : c2802xlib/ePWM  PwmType=C2000_Type4  useModule=ePWM2  ePWMxLINKTBPRD=Not Linked  periodUnits=Clock cycles  timerSource=Specify via dialog  timerPeriod_clk=target.PWM_Counter_Period+1  timerPeriod_sec=0.0001  tbshadow=Counter equals to zero  countingMode=Up-Down  phaseActiveEnable=Set counter to phase value specified via dialog  phaseDirection=Count up after sync  phaseActive=0  synchronizationEnable=off  dcaevt1Sync=off  dcbevt1Sync=off  synchronizationOption=Pass through (EPWMxSYNCI or SWFSYNC)  perSynchronizationOption=Counter equals to period (CTR=PRD)  clockPrescale=1  HSclockPrescale=1  enswap=off  ePWMxAStatus=on  ePWMxAactionLogic1=Do nothing  ePWMxAactionLogic2=Do nothing  ePWMxAactionLogic3=Clear  ePWMxAactionLogic4=Set  ePWMxAactionLogic5=Do nothing  ePWMxAactionLogic6=Do nothing  ePWMxACSFenable=off  ePWMxACSFvalue=Forcing disable  ePWMxASFreload=Zero  ePWMxBStatus=off  ePWMxBactionLogic1=Set  ePWMxBactionLogic2=Clear  ePWMxBactionLogic3=Do nothing  ePWMxBactionLogic4=Do nothing  ePWMxBactionLogic5=Clear  ePWMxBactionLogic6=Set  ePWMxBCSFenable=off  ePWMxBCSFvalue=Forcing disable  ePWMxBSFreload=Zero  ePWNxBOutWay=off  ePWMxLINKCMPA=Not Linked  CMPAUnits=Clock cycles  CMPASource=Input port  CMPAValue_per=50  CMPAValue_clk=floor(target.PWM_Counter_Period/2+1)  enCMPAshadow=Counter equals to zero (CTR=Zero)  ePWMxLINKCMPB=Not Linked  CMPBUnits=Clock cycles  CMPBSource=Specify via dialog  CMPBValue_per=50  CMPBValue_clk=floor(target.PWM_Counter_Period/2+1)  enCMPBshadow=Counter equals to zero (CTR=Zero)  ePWMxLINKCMPC=Not Linked  CMPCUnits=Clock cycles  CMPCSource=Specify via dialog  CMPCValue_per=50  CMPCValue_clk=32000  enCMPCshadow=Counter equals to zero (CTR=Zero)  ePWMxLINKCMPD=Not Linked  CMPDUnits=Clock cycles  CMPDSource=Specify via dialog  CMPDValue_per=50  CMPDValue_clk=32000  enCMPDshadow=Counter equals to zero (CTR=Zero)  enableDBePWMxA=on  enableDBePWMxB=on  enhalfcycle=off  DBpolarity=Active high complementary (AHC)  DBedgeDelay=Positive  DBSource_ePWMxA=ePWMxA  DBSource_ePWMxB=ePWMxA  DBPeriodUnits=Clock cycles  DBperiodSource=Specify via dialog  REDperiod=15  FEDperiod=15  REDperiod_sec=0  FEDperiod_sec=0  LoadModeDBRED=Immediate without using shadow  LoadModeDBFED=Immediate without using shadow  adcstartModuleA=off  adcrequestEventA=First event  adcstartEventA=Digital Compare Module A Event 1 start of conversion (DCAEVT1.soc)  adcstartEventA_type2=Counter equals to period (CTR=PRD)  adcstartModuleB=off  adcrequestEventB=First event  adcstartEventB=Counter equals to zero (CTR=Zero)  adcstartEventB_type2=Counter equals to zero (CTR=Zero)  intEn=off  intPrd=First event  intSel=Counter equals to zero (CTR=Zero)  intSel_type2=Counter equals to zero (CTR=Zero)  hrpe=off  enHRPWM=off  HRPWM_LoadMode=Counter equals to period (CTR=PRD)  HRPWM_CTLMode=Duty or Period control mode  HRPWM_EDGMode=Both edge  hrpeb=off  enHRPWMB=off  HRPWM_LoadModeB=Counter equals to zero (CTR=ZERO)  HRPWM_CTLModeB=Duty or Period control mode  HRPWM_EDGModeB=Both edge  enHRDBRED=off  enHRDBFED=off  enSFO=on  enautoconv=on  chopperEnable=off  chopperFrequency=1  chopperFirstwidth=1  chopperDuty=12.5%  tripZonesource=Specify via dialog  tzselOSHT1=off  tzselOSHT2=off  tzselOSHT3=off  tzselOSHDCAEV1=off  tzselOSHDCBEV1=off  tzselCBC1=off  tzselCBC2=off  tzselCBC3=off  tzselCBCDCAEV2=off  tzselCBCDCBEV2=off  tzselOSHT4=off  tzselOSHT5=off  tzselOSHT6=off  tzselCBC4=off  tzselCBC5=off  tzselCBC6=off  enTzOstIntr=off  enTzCbcIntr=off  enTzDCAEVT1Intr=off  enTzDCAEVT2Intr=off  enTzDCBEVT1Intr=off  enTzDCBEVT2Intr=off  ePWMxAforced=No action  ePWMxBforced=No action  DCAEVT1forced=No action  DCBEVT1forced=No action  DCAEVT2forced=No action  DCBEVT2forced=No action  dcah=Trip Zone 1 input (TZ1)  dcal=Trip Zone 2 input (TZ2)  dcbh=Trip Zone 1 input (TZ1)  dcbl=Trip Zone 2 input (TZ2)  dcah_type2=GPTRIP1SEL/(TZ1)  dcal_type2=GPTRIP2SEL/(TZ2)  dcbh_type2=GPTRIP1SEL/(TZ1)  dcbl_type2=GPTRIP2SEL/(TZ2)  gendcaevt1=Event disabled  gendcaevt2=Event disabled  gendcbevt1=Event disabled  gendcbevt2=Event disabled  dcaevt1src=DCAEVT1 with sync  dcaevt2src=DCAEVT2 with sync  dcbevt1src=DCBEVT1 with sync  dcbevt2src=DCBEVT2 with sync  pulsesel=Counter equals to zero (CTR=Zero)  blankinv=off  blankoffset=0  blankwidth=0  evsrcsel=Filtered version of DCAEVT1 (DCAEVT1FILT)  encape=off
  wires:
  Data Store Read/1 -> Switch4/2, Switch1/2
  Constant2/1 -> Switch4/3
  dutyA/1 -> Sum/1, Switch4/1
  Switch4/1 -> ePWM1/1
  Switch1/1 -> ePWM2/1
  Sum/1 -> Switch1/1
  PWM_Counter_Period/1 -> Sum/2
  Constant1/1 -> Switch1/3

== system mod_firmware_NVH_v6/State Machine/ERROR, POWER_OFF, POWER_ON ==
  Enable : EnablePort  StatesWhenEnabling=reset
  Constant : Constant  Value=0  OutDataTypeStr=boolean  SampleTime=Tref
  Constant1 : Constant  Value=0  OutDataTypeStr=single  SampleTime=Tref
  Constant2 : Constant  Value=0  OutDataTypeStr=boolean  SampleTime=Tref
  Data Store Write1 : DataStoreWrite  DataStoreName=slowPID  IndexOptions=Index vector (dialog)  Indices=1  OutputSizes=1
  Data Store Write6 : DataStoreWrite  DataStoreName=control_en  IndexOptions=Index vector (dialog)  Indices=1  OutputSizes=1
  pos_ref : Outport
  wires:
  Constant/1 -> Data Store Write6/1
  Constant1/1 -> pos_ref/1
  Constant2/1 -> Data Store Write1/1

== system mod_firmware_NVH_v6/State Machine/POSITIONING ==
  Enable : EnablePort  StatesWhenEnabling=reset
  Constant : Constant  OutDataTypeStr=boolean  SampleTime=Tref
  Constant1 : Constant  OutDataTypeStr=boolean  SampleTime=Tref
  Constant2 : Constant  Value=0  OutDataTypeStr=single  SampleTime=Tref
  Data Store Write1 : DataStoreWrite  DataStoreName=slowPID  IndexOptions=Index vector (dialog)  Indices=1  OutputSizes=1
  Data Store Write6 : DataStoreWrite  DataStoreName=control_en  IndexOptions=Index vector (dialog)  Indices=1  OutputSizes=1
  pos_ref : Outport
  wires:
  Constant2/1 -> pos_ref/1
  Constant1/1 -> Data Store Write1/1
  Constant/1 -> Data Store Write6/1

== system mod_firmware_NVH_v6/State Machine/PROFILE ==
  Enable : EnablePort  StatesWhenEnabling=reset
  Constant : Constant  OutDataTypeStr=boolean  SampleTime=Tref
  Constant1 : Constant  Value=0  OutDataTypeStr=boolean  SampleTime=Tref
  Data Store Write1 : DataStoreWrite  DataStoreName=slowPID  IndexOptions=Index vector (dialog)  Indices=1  OutputSizes=1
  Data Store Write6 : DataStoreWrite  DataStoreName=control_en  IndexOptions=Index vector (dialog)  Indices=1  OutputSizes=1
  Excitation profile : simulink/Sources/Repeating Sequence Stair  OutValues=qint  tsamp=Tref  OutMin=[]  OutMax=[]  OutDataTypeStr=single  OutputDataTypeScalingMode=single  OutDataType=dataType  ConRadixGroup=Best Precision: Vector-wise  OutScaling=[]
  pos_ref : Outport
  wires:
  Constant/1 -> Data Store Write6/1
  Excitation profile/1 -> pos_ref/1
  Constant1/1 -> Data Store Write1/1

== system mod_firmware_NVH_v6/State Machine/RAND_ISO ==
  Enable : EnablePort  StatesWhenEnabling=reset
  Constant : Constant  OutDataTypeStr=boolean  SampleTime=Tref
  Constant1 : Constant  Value=0  OutDataTypeStr=boolean  SampleTime=Tref
  Data Store Write1 : DataStoreWrite  DataStoreName=slowPID  IndexOptions=Index vector (dialog)  Indices=1  OutputSizes=1
  Data Store Write6 : DataStoreWrite  DataStoreName=control_en  IndexOptions=Index vector (dialog)  Indices=1  OutputSizes=1
  Gstroke in mm : DiscreteTransferFcn  NumeratorSource=Input port  Numerator=numz*1000  DenominatorSource=Input port  Denominator=denz  SampleTime=Tref  a0EqualsOne=on
      settings: InputPortMap=u0,p1,p3
  ISO road profile in m : Subsystem
  Subsystem : Subsystem
  pos_ref_mm : Outport
  wires:
  Constant/1 -> Data Store Write6/1
  Constant1/1 -> Data Store Write1/1
  Gstroke in mm/1 -> pos_ref_mm/1
  Subsystem/2(denz) -> Gstroke in mm/3
  ISO road profile in m/1(zroad_m) -> Gstroke in mm/1
  Subsystem/1(numz) -> Gstroke in mm/2

== system mod_firmware_NVH_v6/State Machine/Reference preprocessing ==
  ref_sm : Inport
  Add : Sum
  Custom rate limiter : Subsystem  TreatAsAtomicUnit=on
  Data Store Read2 : DataStoreRead  DataStoreName=pos_meas_mm  SampleTime=Tper  IndexOptions=Index vector (dialog)  Indices=1  OutputSizes=1
  Data Store Read3 : DataStoreRead  DataStoreName=pos_init_mm  SampleTime=Tper  IndexOptions=Index vector (dialog)  Indices=1  OutputSizes=1
  Data Store Read6 : DataStoreRead  DataStoreName=slowPID  SampleTime=Tper  IndexOptions=Index vector (dialog)  Indices=1  OutputSizes=1
  Rate Limiter1 : RateLimiter  RisingSlewLimit=rate_lim  FallingSlewLimit=-rate_lim  SampleTimeMode=inherited
  Saturation : Saturate  UpperLimit=22  LowerLimit=-22
  Switch : Switch  Criteria=u2 > Threshold  SaturateOnIntegerOverflow=off  InputSameDT=off
  pos_ref_mm : Outport
  wires:
  Data Store Read6/1 -> Switch/2, Custom rate limiter/Enable
  ref_sm/1 -> Add/2
  Data Store Read3/1 -> Custom rate limiter/1(u), Rate Limiter1/1
  Rate Limiter1/1 -> Add/1
  Saturation/1 -> pos_ref_mm/1
  Data Store Read2/1 -> Custom rate limiter/2(x0)
  Custom rate limiter/1(Y) -> Switch/1
  Add/1 -> Switch/3
  Switch/1 -> Saturation/1

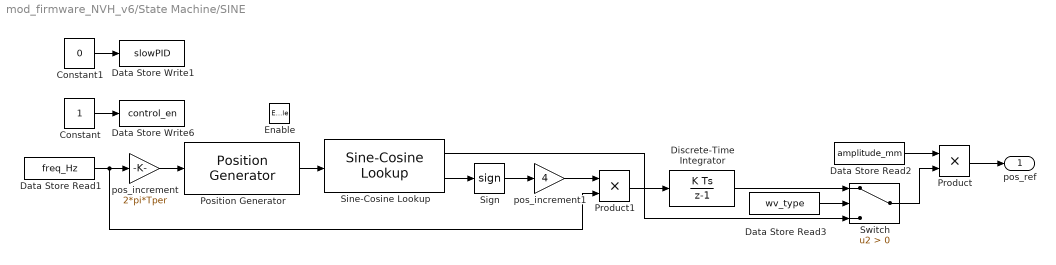
== system mod_firmware_NVH_v6/State Machine/SINE ==
  Enable : EnablePort  StatesWhenEnabling=reset
  Constant : Constant  OutDataTypeStr=boolean  SampleTime=Tper
  Constant1 : Constant  Value=0  OutDataTypeStr=boolean  SampleTime=Tper
  Data Store Read1 : DataStoreRead  DataStoreName=freq_Hz  SampleTime=Tper  IndexOptions=Index vector (dialog)  Indices=1  OutputSizes=1
  Data Store Read2 : DataStoreRead  DataStoreName=amplitude_mm  SampleTime=Tper  IndexOptions=Index vector (dialog)  Indices=1  OutputSizes=1
  Data Store Read3 : DataStoreRead  DataStoreName=wv_type  SampleTime=Tper  IndexOptions=Index vector (dialog)  Indices=1  OutputSizes=1
  Data Store Write1 : DataStoreWrite  DataStoreName=slowPID  IndexOptions=Index vector (dialog)  Indices=1  OutputSizes=1
  Data Store Write6 : DataStoreWrite  DataStoreName=control_en  IndexOptions=Index vector (dialog)  Indices=1  OutputSizes=1
  Discrete-Time Integrator : DiscreteIntegrator  SampleTime=-1  LimitOutput=on  UpperSaturationLimit=1  LowerSaturationLimit=-1  ICPrevOutput=DiscIntNeverNeededParam  ICPrevScaledInput=DiscIntNeverNeededParam
  Position Generator : mcbcontrolslib/Position Generator  AngleOutput=Radians  ThetaSource=External  ThetaInput=5e-4  DataType=double  ExternalReset=none  Offset=0
      settings: SourceProductBaseCode=MT
  Product : Product
  Product1 : Product
  Sign : Signum
  Sine-Cosine Lookup : mcbcontrolslib/Sine-Cosine Lookup  AngleInput=Radians  N_points=1024
      settings: SourceProductBaseCode=MT
  Switch : Switch  Criteria=u2 > Threshold  SaturateOnIntegerOverflow=off  InputSameDT=off
  pos_increment : Gain  Gain=2*pi*Tper  RndMeth=Simplest  OutDataTypeStr=Inherit: Same as input
  pos_increment1 : Gain  Gain=4  RndMeth=Simplest  OutDataTypeStr=Inherit: Same as input
  pos_ref : Outport
  wires:
  Constant/1 -> Data Store Write6/1
  pos_increment/1 -> Position Generator/1
  Position Generator/1 -> Sine-Cosine Lookup/1
  Sine-Cosine Lookup/2 -> Sign/1
  Data Store Read2/1 -> Product/1
  Data Store Read1/1 -> Product1/2, pos_increment/1
  Product/1 -> pos_ref/1
  Constant1/1 -> Data Store Write1/1
  Sign/1 -> pos_increment1/1
  Discrete-Time Integrator/1 -> Switch/1
  Sine-Cosine Lookup/1 -> Switch/3
  Data Store Read3/1 -> Switch/2
  Switch/1 -> Product/2
  Product1/1 -> Discrete-Time Integrator/1
  pos_increment1/1 -> Product1/1
